simulink model "week3_problem2"  (R2020b)
settings: Solver=VariableStepAuto  StartTime=0.0  StopTime=10  RelTol=1e-3
settings Model: Creator=gokul  LastModifiedBy=gokul

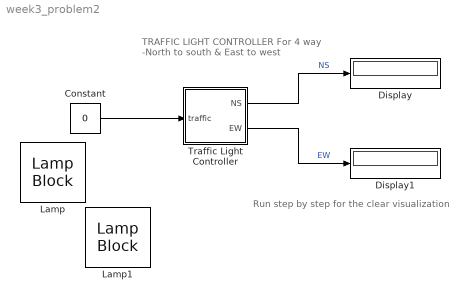
== system week3_problem2 ==
  note: Run step by step for the clear visualization
  note: TRAFFIC LIGHT CONTROLLER
      | For 4 way -North to south & East to west
  Constant : Constant  Value=0
  Display : Display
  Display1 : Display
  Lamp : LampBlock
  Lamp1 : LampBlock
  Traffic Light Controller : Stateflow chart  TreatAsAtomicUnit=on
  wires:
  Constant/1 -> Traffic Light Controller/1(traffic)
  Traffic Light Controller/2(EW) -> Display1/1  "EW"
  Traffic Light Controller/1(NS) -> Display/1  "NS"

== stateflow chart week3_problem2/Traffic Light Controller ==
  state Stop
    entry:
    NS=1;
    EW=3;
  state Start_to_go
    entry:
    NS=2;
    EW=1;
  state go
    entry:
    NS=3;
    EW=1;
  state start_to_stop
    entry:
    NS=2;
    EW=1;
  (default) -> Stop
  Stop -> Start_to_go : [traffic==0]{after(100,tick);}
  Start_to_go -> go : [traffic==0]{after(30,tick);}
  start_to_stop -> Stop : [traffic==0]{after(100,tick);}
  go -> start_to_stop : [traffic==0]{after(200,tick);}
  data: NS output =1; EW output =3; traffic input
